simulink model "BPiKU_v3"  (R2018b)
settings: Solver=ode23t  StartTime=0.0  StopTime=6  RelTol=1e-6
undefined symbols (not defined in the file): Cdc, i_kt_int, i_kt_p, LdM, Lout, PointsVAH_I, PointsVAH_U, Rd, RdM, sigbuilder_block, u_k_int, u_k_p
libraries: powerlib x45, simulink x7, powerlib_meascontrol x3
settings Model: SimulationMode=accelerator  Creator=K2  LastModifiedBy=K2

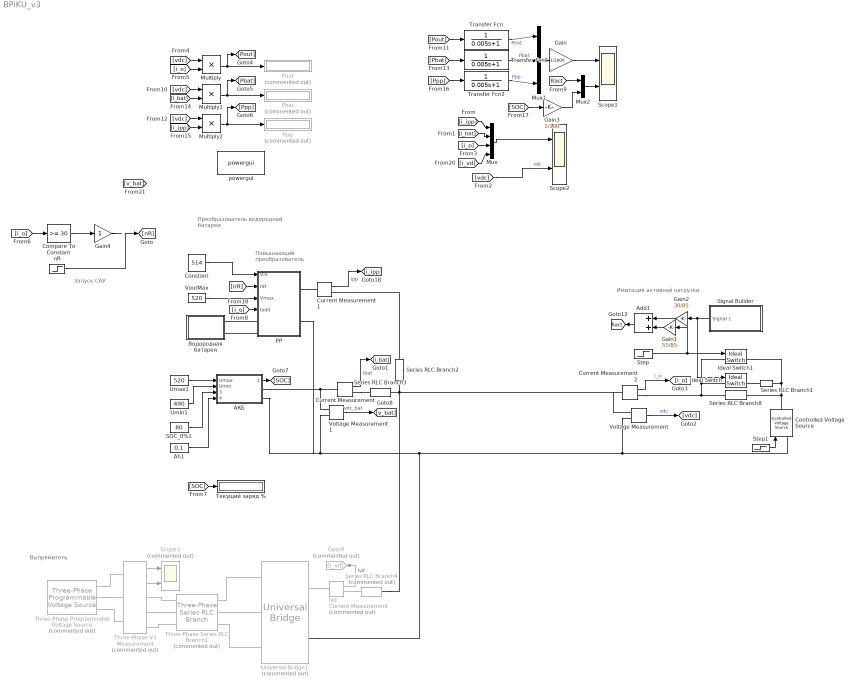
== system BPiKU_v3 ==
  note: Повышающий
      | преобразователь
  note: Имитация активной нагрузки
  note: Преобразователь водородной батареи
  note: Запуск САУ
  note: Выпрямитель
  Add1 : Sum
  Ah1 : Constant  Value=0.1
  Compare To Constant : simulink/Logic and Bit Operations/Compare To Constant  relop=>=  const=30  OutDataTypeStr=boolean
  Constant : Constant  Value=514
  Controlled Voltage Source : powerlib/Electrical Sources/Controlled Voltage Source  Initialize=on  Source_Type=AC  Amplitude=0  Phase=0  Frequency=0  Measurements=None
  Current Measurement : powerlib/Measurements/Current Measurement  PhasorSimulation=off  OutputType=Complex  PSBequivalent=0
  Current Measurement1 : powerlib/Measurements/Current Measurement  PhasorSimulation=off  OutputType=Complex  PSBequivalent=0
  Current Measurement2 : powerlib/Measurements/Current Measurement  PhasorSimulation=off  OutputType=Complex  PSBequivalent=0
  Gain : Gain  Gain=1/1000
  Gain1 : Gain  Gain=55/85
  Gain2 : Gain  Gain=30/85
  Gain3 : Gain  Gain=1/100
  Gain4 : Gain  OutDataTypeStr=double
  Goto9 : Goto  Commented=on  GotoTag=i_vd
  Ideal Switch : powerlib/Power Electronics/Ideal Switch  Ron=510*510/30000  Lon=0  IC=0  Rs=1e5  Cs=inf  Measurements=on
  Ideal Switch1 : powerlib/Power Electronics/Ideal Switch  Ron=550*550/45000  Lon=0  IC=0  Rs=1e5  Cs=inf  Measurements=on
  Multiply : Product
  Multiply1 : Product
  Multiply2 : Product
  Mux : Mux
  Mux1 : Mux  Inputs=3
  Mux2 : Mux  Inputs=2
  PP : Subsystem
  Pbat : Display  Commented=on
      settings: Format=bank
  Pout : Display  Commented=on
      settings: Format=bank
  Ppp : Display  Commented=on
      settings: Format=bank
  SOC_0%1 : Constant  Value=80
  Scope1 : Scope  NumInputPorts=2
  Scope2 : Scope  NumInputPorts=2
  Scope3 : Scope  Commented=on  NumInputPorts=2
  Series RLC Branch1 : powerlib/Elements/Series RLC Branch  LConnTagsString=__new0  RConnTagsString=__new0  BranchType=L  Resistance=550/130  Inductance=10e-3  SetiL0=off  InitialCurrent=0  Capacitance=1000e-6  Setx0=off  InitialVoltage=0  Measurements=None
  Series RLC Branch2 : powerlib/Elements/Series RLC Branch  LConnTagsString=__new0  RConnTagsString=__new0  BranchType=R  Resistance=0.01  Inductance=10e-6  SetiL0=off  InitialCurrent=0  Capacitance=1000e-6  Setx0=off  InitialVoltage=0  Measurements=None
  Series RLC Branch3 : powerlib/Elements/Series RLC Branch  LConnTagsString=__new0  RConnTagsString=__new0  BranchType=R  Resistance=0.01  Inductance=10e-6  SetiL0=off  InitialCurrent=0  Capacitance=1000e-6  Setx0=off  InitialVoltage=0  Measurements=None
  Series RLC Branch4 : powerlib/Elements/Series RLC Branch  Commented=on  LConnTagsString=__new0  RConnTagsString=__new0  BranchType=R  Resistance=0.01  Inductance=10e-6  SetiL0=off  InitialCurrent=0  Capacitance=1000e-6  Setx0=off  InitialVoltage=0  Measurements=None
  Series RLC Branch8 : powerlib/Elements/Series RLC Branch  LConnTagsString=__new0  RConnTagsString=__new0  BranchType=Open circuit  Resistance=550/130  Inductance=10e-6  SetiL0=off  InitialCurrent=0  Capacitance=1000e-6  Setx0=off  InitialVoltage=0  Measurements=None
  Signal Builder : Subsystem  Tag=STV Subsys  LoadFcn=sigbuilder_block('load');  StartFcn=sigbuilder_block('start');  StopFcn=sigbuilder_block('stop');  ClipboardFcn=sigbuilder_block('clipboard');  mask(Sigbuilder block){tuvar=[0:10]}
      mask help: Simulink:masks:SigbuilderBlock_MD
      mask init:
      | if ~strcmp(get_param(bdroot(gcbh),'SimulationStatus'),'stopped') tuvar = sigbuilder_block('maskInit'); end
      settings: CopyFcn=sigbuilder_block('copy');  DeleteFcn=sigbuilder_block('delete');  ModelCloseFcn=sigbuilder_block('modelClose');  PreSaveFcn=sigbuilder_block('preSave');  PauseFcn=sigbuilder_block('pause');  ContinueFcn=sigbuilder_block('continue');  NameChangeFcn=sigbuilder_block('namechange');  OpenFcn=sigbuilder_block('open',[193.5 84.75 550.5 399.75 ]);  CloseFcn=sigbuilder_block('close');
      mask Display: plot(0, 0, 100, 100,[2, 2, 32, 32, 2], [68, 8, 8, 68, 68],[32, 2], [38, 38], [32, 19, 2],[53, 60, 44], [32, 17, 17, 2],[16, 16, 31, 31]);txt = getActiveGroup(gcbh);text(2, 100, txt,'verticalAlignment', 'top');
  Step : Step  Time=4  SampleTime=0
  Step1 : Step  Time=3.5  After=800*0  SampleTime=0
  Three-Phase Programmable Voltage Source : powerlib/Electrical Sources/Three-Phase Programmable Voltage Source  Commented=on  PositiveSequence="[400  0 50]"  VariationEntity=None  VariationType=Table of time-amplitude pairs  VariationTypeAlt=Step  VariationStep=0.5  VariationRate=10  VariationMagnitude=0.3  VariationFrequency=2  VariationTiming=[1 2]  VariationPhaseA=off  Amplitudes=[1 0.8 1.2 1.0]  TimeValues=[0 0.1 0.15 0.2]  HarmonicGeneration=off  HarmonicA=[3 0.2 -25 0]  HarmonicB=[2 0.15 35 2]  Timing="[0.05  3]"  BusType=swing  Pref=0  Qref=0  Qmin=-inf  Qmax=inf
  Three-Phase Series RLC Branch1 : powerlib/Elements/Three-Phase Series RLC Branch  Commented=on  LConnTagsString=A|B|C  RConnTagsString=A|B|C  BranchType=RL  Resistance=0.001  Inductance=250e-6  Capacitance=105e-6  Measurements=None
  Three-Phase V-I Measurement : powerlib/Measurements/Three-Phase V-I Measurement  Commented=on  VoltageMeasurement=phase-to-phase  SetLabelV=off  LabelV=Vabc  Vpu=off  VpuLL=off  CurrentMeasurement=yes  SetLabelI=off  LabelI=Iabc  Ipu=off  Pbase=100e6  Vbase=500e3  OutputType=Complex  PhasorSimulation=off  PSBequivalent=0
  Transfer Fcn : TransferFcn  Denominator=[0.005 1]
  Transfer Fcn1 : TransferFcn  Denominator=[0.005 1]
  Transfer Fcn2 : TransferFcn  Denominator=[0.005 1]
  Umax1 : Constant  Value=520
  Umin1 : Constant  Value=490
  Universal Bridge1 : powerlib/Power Electronics/Universal Bridge  Commented=on  Arms=3  SnubberResistance=1e5  SnubberCapacitance=inf  Device=Diodes  Ron=1e-3  Lon=0  ForwardVoltages="[  0  0  ]"  ForwardVoltage=0  GTOparameters=[ 10e-6 , 20e-6 ]  IGBTparameters=[ 1e-6 , 2e-6 ]  Measurements=None  Measurements_2=None  converterType=Rectifier
  Voltage Measurement : powerlib/Measurements/Voltage Measurement  PhasorSimulation=off  OutputType=Complex  PSBequivalent=0
  Voltage Measurement1 : powerlib/Measurements/Voltage Measurement  PhasorSimulation=off  OutputType=Complex  PSBequivalent=0
  VoutMax : Constant  Value=520  SampleTime=0
  ivd : powerlib/Measurements/Current Measurement  Commented=on  PhasorSimulation=off  OutputType=Complex  PSBequivalent=0
  nR : Step  Time=0  SampleTime=1.5/freq/2
  powergui : powerlib/powergui  Priority=1  SimulationMode=Discrete  SampleTime=1e-6  frequency=60  Iterations=50  frequencyindice=0  Pbase=100e6  ErrMax=1e-4  UnitsV=kV  UnitsW=MW  buscounter=0  FunctionMessages=off  echomessages=off  EnableUseOfTLC=off  CurrentSourceSwitches=off  DisableSnubberDevices=off  DisableRonSwitches=off  DisableVfSwitches=off  DisplayEquations=off  SolverType=Tustin  Interpol=off  ExternalGateDelay=off  methode=off  Ts=100  x0status=blocks  SPID=off  SwTol=0  HookPort=off  RestoreLinks=warning  ResistiveCurrentMeasurement=off  Frange=[0:2:500]  Ylog=off  Xlog=on  ShowGrid=off  save=off  variable=ZData  structure=0  ZoomFFT=off  StartTime=0.0  cycles=1  DisplayStyle=1  fundamental=60  FreqAxis=off  MaxFrequency=1000  frequencyindicesteady=1  RmsSteady=1  display=off
  АКБ : Subsystem
  Водородная батарея : Subsystem
  Текущий заряд % : Display
      settings: Format=bank
  tag scope: Ract=global
  wires:
  Signal Builder/1(Signal 1) -> Gain2/1, Ideal Switch/1
  VoutMax/1 -> PP/3(Vmax)
  [nR] -> PP/2(nR)
  Current Measurement1/1 -> [i_ipp]  "ipp"
  [vdc] -> Scope2/2  "vdc"
  Mux/1 -> Scope2/1
  [i_ipp] -> Mux/1
  Current Measurement/1 -> [i_bat]  "ibat"
  [i_bat] -> Mux/2
  Voltage Measurement/1 -> [vdc]  "vdc"
  Current Measurement2/1 -> [i_o]  "i_o"
  [i_o] -> Mux/3
  [vdc] -> Multiply/1
  [i_o] -> Multiply/2
  Multiply/1 -> [Pout], Pout/1
  Step/1 -> Ideal Switch1/1, Gain1/1
  [Ppp] -> Transfer Fcn2/1
  [Pbat] -> Transfer Fcn1/1
  [Pout] -> Transfer Fcn/1
  [vdc] -> Multiply1/1
  [i_bat] -> Multiply1/2
  [i_ipp] -> Multiply2/2
  [vdc] -> Multiply2/1
  Multiply1/1 -> [Pbat], Pbat/1
  Multiply2/1 -> [Ppp], Ppp/1
  Transfer Fcn/1 -> Mux1/1  "Pout"
  Transfer Fcn1/1 -> Mux1/2  "Pbat"
  Transfer Fcn2/1 -> Mux1/3  "Ppp"
  АКБ/1(CurSOC%) -> [SOC]
  [SOC] -> Текущий заряд %/1
  Constant/1 -> PP/1(Vin)
  Mux1/1 -> Gain/1
  [Ract] -> Mux2/1
  Gain/1 -> Scope1/1
  Add1/1 -> [Ract]
  Gain1/1 -> Add1/2
  Gain2/1 -> Add1/1
  Mux2/1 -> Scope1/2
  [SOC] -> Gain3/1
  Gain3/1 -> Mux2/2
  Compare To Constant/1 -> Gain4/1
  Three-Phase V-I Measurement/2 -> Scope3/2
  Three-Phase V-I Measurement/1 -> Scope3/1
  ivd/1 -> Goto9/1  "ivd"
  [i_vd] -> Mux/4
  Step1/1 -> Controlled Voltage Source/1
  SOC_0%1/1 -> АКБ/3(InitSOC%)
  Umax1/1 -> АКБ/1(Umax)
  Ah1/1 -> АКБ/4(CapMaxAh)
  Umin1/1 -> АКБ/2(Umin)
  [i_o] -> Compare To Constant/1
  nR/1 -> [nR]
  Gain4/1 -> ?
  [i_o] -> PP/4(Iadd)
  Voltage Measurement1/1 -> [v_bat]  "vdc_bat"
  connections:
  Ideal Switch/RConn1 -- Series RLC Branch1/LConn1
  PP/LConn2 -- Водородная батарея/RConn2
  PP/LConn1 -- Водородная батарея/RConn1
  PP/RConn1 -- Current Measurement1/LConn1
  Series RLC Branch8/LConn1 -- Current Measurement2/RConn1 -- Ideal Switch/LConn1 -- Ideal Switch1/LConn1
  Series RLC Branch2/LConn1 -- Current Measurement1/RConn1
  Current Measurement/RConn1 -- Series RLC Branch3/RConn1
  Voltage Measurement/LConn2 -- Voltage Measurement1/LConn2 -- PP/RConn2 -- АКБ/RConn2 -- Universal Bridge1/RConn2 -- Controlled Voltage Source/LConn1
  Universal Bridge1/LConn3 -- Three-Phase Series RLC Branch1/RConn3
  Three-Phase Series RLC Branch1/RConn2 -- Universal Bridge1/LConn2
  Three-Phase Programmable Voltage Source/RConn2 -- Three-Phase V-I Measurement/LConn2
  Three-Phase Programmable Voltage Source/RConn3 -- Three-Phase V-I Measurement/LConn3
  Universal Bridge1/LConn1 -- Three-Phase Series RLC Branch1/RConn1
  Three-Phase Programmable Voltage Source/RConn1 -- Three-Phase V-I Measurement/LConn1
  ivd/LConn1 -- Universal Bridge1/RConn1
  Series RLC Branch4/RConn1 -- ivd/RConn1
  Series RLC Branch3/LConn1 -- Current Measurement2/LConn1 -- Voltage Measurement/LConn1 -- Series RLC Branch4/LConn1 -- Series RLC Branch2/RConn1
  Three-Phase Series RLC Branch1/LConn3 -- Three-Phase V-I Measurement/RConn3
  Three-Phase Series RLC Branch1/LConn2 -- Three-Phase V-I Measurement/RConn2
  Three-Phase Series RLC Branch1/LConn1 -- Three-Phase V-I Measurement/RConn1
  Ideal Switch1/RConn1 -- Series RLC Branch1/RConn1 -- Series RLC Branch8/RConn1 -- Controlled Voltage Source/RConn1
  АКБ/RConn1 -- Voltage Measurement1/LConn1 -- Current Measurement/LConn1

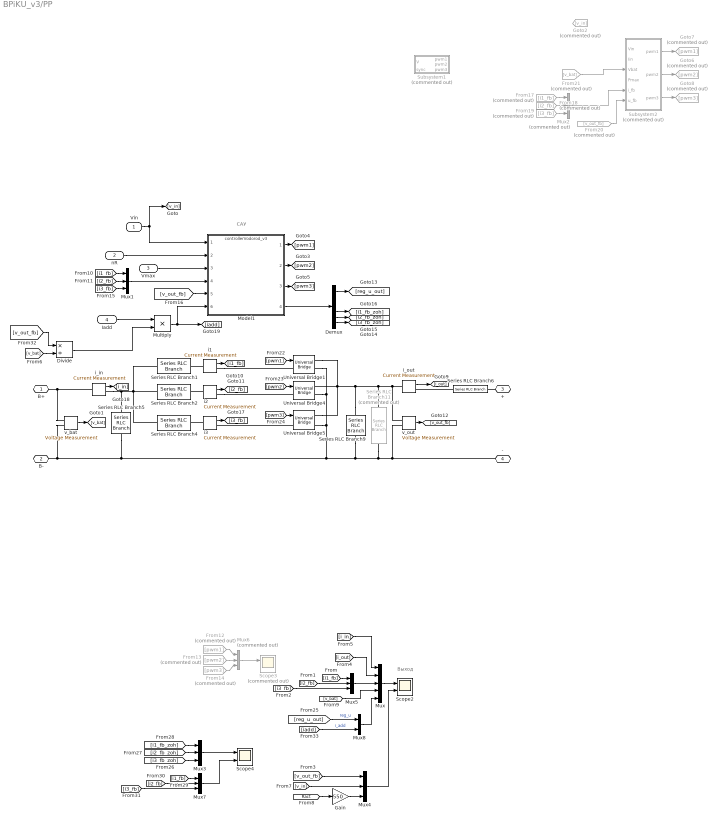
== system BPiKU_v3/PP ==
  note: САУ
  note: Выход
  Vin : Inport
  nR : Inport  Port=2
  Vmax : Inport  Port=3
  Iadd : Inport  Port=4
  Demux : Demux  Outputs=7
  Divide : Product  Inputs=*/
  From12 : From  Commented=on  GotoTag=pwm1
  From13 : From  Commented=on  GotoTag=pwm2
  From14 : From  Commented=on  GotoTag=pwm3
  From17 : From  Commented=on  GotoTag=i1_fb
  From18 : From  Commented=on  GotoTag=i2_fb
  From19 : From  Commented=on  GotoTag=i3_fb
  From20 : From  Commented=on  GotoTag=v_out_fb
  From21 : From  Commented=on  GotoTag=v_bat
  Gain : Gain  Gain=550
  Goto2 : Goto  Commented=on  GotoTag=v_in
  Goto6 : Goto  Commented=on  GotoTag=pwm2
  Goto7 : Goto  Commented=on  GotoTag=pwm1
  Goto8 : Goto  Commented=on  GotoTag=pwm3
  Model1 : ModelReference  ModelNameDialog=controllerVodorod_v3.slx  SimulationMode=Normal  ModelReferenceVersion=1.32
  Multiply : Product
  Mux : Mux  Inputs=5
  Mux{1,3..5,7} (5 alike) : Mux  Inputs=3
  Mux2 : Mux  Commented=on  Inputs=3
  Mux6 : Mux  Commented=on  Inputs=3
  Mux8 : Mux  Inputs=2
  Scope2 : Scope  NumInputPorts=2
  Scope3 : Scope  Commented=on  NumInputPorts=2
  Scope4 : Scope  NumInputPorts=2
  Series RLC Branch1 : powerlib/Elements/Series RLC Branch  LConnTagsString=__new0  RConnTagsString=__new0  BranchType=RL  Resistance=RdM(1)  Inductance=LdM(1)  SetiL0=off  InitialCurrent=0  Capacitance=100e-6  Setx0=off  InitialVoltage=0  Measurements=None
  Series RLC Branch11 : powerlib/Elements/Series RLC Branch  Commented=on  LConnTagsString=__new0  RConnTagsString=__new0  BranchType=Open circuit  Resistance=2000  Inductance=50e-6  SetiL0=off  InitialCurrent=0  Capacitance=100e-6  Setx0=off  InitialVoltage=0  Measurements=None
  Series RLC Branch2 : powerlib/Elements/Series RLC Branch  LConnTagsString=__new0  RConnTagsString=__new0  BranchType=RL  Resistance=RdM(2)  Inductance=LdM(2)  SetiL0=off  InitialCurrent=0  Capacitance=100e-6  Setx0=off  InitialVoltage=0  Measurements=None
  Series RLC Branch4 : powerlib/Elements/Series RLC Branch  LConnTagsString=__new0  RConnTagsString=__new0  BranchType=RL  Resistance=RdM(3)  Inductance=LdM(3)  SetiL0=off  InitialCurrent=0  Capacitance=100e-6  Setx0=off  InitialVoltage=0  Measurements=None
  Series RLC Branch5 : powerlib/Elements/Series RLC Branch  LConnTagsString=__new0  RConnTagsString=__new0  BranchType=RC  Resistance=0.001  Inductance=50e-6  SetiL0=off  InitialCurrent=0  Capacitance=8000e-6  Setx0=on  InitialVoltage=340  Measurements=None
  Series RLC Branch6 : powerlib/Elements/Series RLC Branch  LConnTagsString=__new0  RConnTagsString=__new0  BranchType=RL  Resistance=Rd  Inductance=Lout  SetiL0=off  InitialCurrent=0  Capacitance=1e-6  Setx0=off  InitialVoltage=0  Measurements=None
  Series RLC Branch9 : powerlib/Elements/Series RLC Branch  LConnTagsString=__new0  RConnTagsString=__new0  BranchType=C  Resistance=0.0001  Inductance=50e-6  SetiL0=off  InitialCurrent=0  Capacitance=Cdc  Setx0=on  InitialVoltage=510  Measurements=None
  Subsystem1 : Subsystem  Commented=on
  Subsystem2 : Subsystem  Commented=on
  Universal Bridge1 : powerlib/Power Electronics/Universal Bridge  Arms=1  SnubberResistance=1e5  SnubberCapacitance=inf  Device=MOSFET / Diodes  Ron=1e-3  Lon=0  ForwardVoltages="[  2  2  ]"  ForwardVoltage=0  GTOparameters=[ 10e-6 , 20e-6 ]  IGBTparameters=[ 1e-6 , 2e-6 ]  Measurements=None  Measurements_2=None  converterType=Rectifier
  Universal Bridge4 : powerlib/Power Electronics/Universal Bridge  Arms=1  SnubberResistance=1e5  SnubberCapacitance=inf  Device=MOSFET / Diodes  Ron=1e-3  Lon=0  ForwardVoltages="[  2  2  ]"  ForwardVoltage=0  GTOparameters=[ 10e-6 , 20e-6 ]  IGBTparameters=[ 1e-6 , 2e-6 ]  Measurements=None  Measurements_2=None  converterType=Rectifier
  Universal Bridge5 : powerlib/Power Electronics/Universal Bridge  Arms=1  SnubberResistance=1e5  SnubberCapacitance=inf  Device=MOSFET / Diodes  Ron=1e-3  Lon=0  ForwardVoltages="[  2  2  ]"  ForwardVoltage=0  GTOparameters=[ 10e-6 , 20e-6 ]  IGBTparameters=[ 1e-6 , 2e-6 ]  Measurements=None  Measurements_2=None  converterType=Rectifier
  i1 : powerlib/Measurements/Current Measurement  PhasorSimulation=off  OutputType=Complex  PSBequivalent=0
  i2 : powerlib/Measurements/Current Measurement  PhasorSimulation=off  OutputType=Complex  PSBequivalent=0
  i3 : powerlib/Measurements/Current Measurement  PhasorSimulation=off  OutputType=Complex  PSBequivalent=0
  i_in : powerlib/Measurements/Current Measurement  PhasorSimulation=off  OutputType=Complex  PSBequivalent=0
  i_out : powerlib/Measurements/Current Measurement  PhasorSimulation=off  OutputType=Complex  PSBequivalent=0
  v_bat : powerlib/Measurements/Voltage Measurement  PhasorSimulation=off  OutputType=Complex  PSBequivalent=0
  v_out : powerlib/Measurements/Voltage Measurement  PhasorSimulation=off  OutputType=Complex  PSBequivalent=0
  B+ : PMIOPort  Side=Left
  B- : PMIOPort  Port=2  Side=Left
  + : PMIOPort  Port=3  Side=Right
  - : PMIOPort  Port=4  Side=Right
  wires:
  From14/1 -> Mux6/3
  From12/1 -> Mux6/1
  [v_in] -> Mux4/2
  Mux5/1 -> Mux/3
  [v_out_fb] -> Mux4/1
  Mux/1 -> Scope2/1
  [i_in] -> Mux/1
  [i_out] -> Mux/2
  [i1_fb] -> Mux5/1
  From13/1 -> Mux6/2
  Mux6/1 -> Scope3/1
  [i2_fb] -> Mux5/2
  Mux4/1 -> Scope2/2
  [i3_fb] -> Mux5/3
  Model1/2 -> [pwm2]
  Model1/1 -> [pwm1]
  Vin/1 -> Model1/1, [v_in]
  Model1/3 -> [pwm3]
  nR/1 -> Model1/2
  Vmax/1 -> Model1/3
  [Ract] -> Gain/1
  Gain/1 -> Mux4/3
  [v_out_fb] -> Model1/5
  [v_bat] -> Mux/4
  [i2_fb] -> Mux1/2
  [i3_fb] -> Mux1/3
  [i1_fb] -> Mux1/1
  Mux1/1 -> Model1/4
  i1/1 -> [i1_fb]
  i_in/1 -> [i_in]
  i_out/1 -> [i_out]
  i2/1 -> [i2_fb]
  v_bat/1 -> [v_bat]
  [pwm1] -> Universal Bridge1/1
  [pwm2] -> Universal Bridge4/1
  v_out/1 -> [v_out_fb]
  [pwm3] -> Universal Bridge5/1
  i3/1 -> [i3_fb]
  From20/1 -> Subsystem2/6(u_fb)
  From21/1 -> Subsystem2/3(Vbat)
  From18/1 -> Mux2/2
  Mux2/1 -> Subsystem2/5(i_fb)
  From17/1 -> Mux2/1
  ? -> Subsystem2/4(Pmax)
  From19/1 -> Mux2/3
  Subsystem2/2(pwm2) -> Goto6/1
  Subsystem2/1(pwm1) -> Goto7/1
  Subsystem2/3(pwm3) -> Goto8/1
  ? -> Subsystem2/2(Iin)
  ? -> Goto2/1, Subsystem2/1(Vin)
  Model1/4 -> Demux/1
  Demux/1 -> [reg_u_out]
  Mux8/1 -> Mux/5
  Demux/7 -> [i3_fb_zoh]
  Demux/6 -> [i2_fb_zoh]
  Demux/5 -> [i1_fb_zoh]
  [i2_fb_zoh] -> Mux3/2
  [i1_fb_zoh] -> Mux3/1
  [i3_fb_zoh] -> Mux3/3
  Mux3/1 -> Scope4/1
  [i2_fb] -> Mux7/2
  [i3_fb] -> Mux7/3
  Mux7/1 -> Scope4/2
  [i1_fb] -> Mux7/1
  Multiply/1 -> [iadd], Model1/6
  Iadd/1 -> Multiply/1
  [v_bat] -> Divide/2
  [v_out_fb] -> Divide/1
  Divide/1 -> Multiply/2
  [reg_u_out] -> Mux8/1  "reg_u"
  [iadd] -> Mux8/2  "i_add"
  connections:
  Series RLC Branch9/LConn1 -- Series RLC Branch11/LConn1 -- v_out/LConn1 -- i_out/LConn1 -- Universal Bridge5/RConn1 -- Universal Bridge1/RConn1 -- Universal Bridge4/RConn1
  v_bat/LConn2 -- B-/RConn1 -- Series RLC Branch5/RConn1 -- Universal Bridge5/RConn2 -- Universal Bridge1/RConn2 -- Universal Bridge4/RConn2 -- Series RLC Branch9/RConn1 -- Series RLC Branch11/RConn1 -- v_out/LConn2 -- -/RConn1
  Series RLC Branch1/LConn1 -- i_in/RConn1 -- Series RLC Branch5/LConn1 -- Series RLC Branch4/LConn1 -- Series RLC Branch2/LConn1
  v_bat/LConn1 -- B+/RConn1 -- i_in/LConn1
  i2/LConn1 -- Series RLC Branch2/RConn1
  +/RConn1 -- Series RLC Branch6/LConn1
  i1/RConn1 -- Universal Bridge1/LConn1
  Series RLC Branch6/RConn1 -- i_out/RConn1
  i2/RConn1 -- Universal Bridge4/LConn1
  Universal Bridge5/LConn1 -- i3/RConn1
  i1/LConn1 -- Series RLC Branch1/RConn1
  i3/LConn1 -- Series RLC Branch4/RConn1

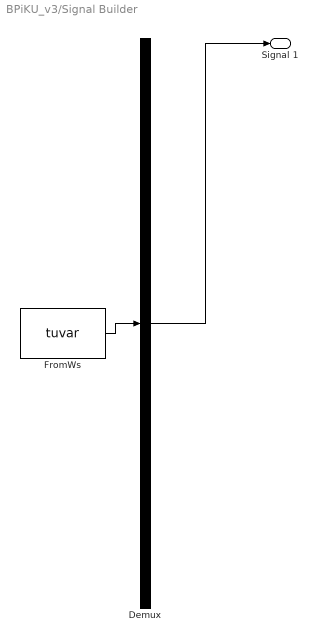
== system BPiKU_v3/Signal Builder ==
  Demux : Demux  Tag=STV Demux  Outputs=1
  FromWs : FromWorkspace  Tag=STV FromWs  VariableName=tuvar  SampleTime=0
      SigBuilderData=|
      | common.afterFinalStr = 'Extrapolate'
      | common.sampleTime = 0
      | dataSet.timeRange = [0 10]
      | dataSet.name = 'Group 1'
      | sbobj.Groups.Name = 'Group 1'
      | sbobj.Groups.Signals.Name = 'Signal 1'
      | sbobj.Groups.Signals.XData = [0 0.02 0.1 0.1 0.17 0.17 0.55 0.55 2.02 2.02 2.07 2.07 2.49 2.49 2.62 2.62 2.87 2.87 3.8 3.8 4.06 4.06 6 10]
      | sbobj.Groups.Signals.YData = [0 0 0 1 1 0 0 1 1 0 0 1 1 0 0 1 1 0 0 1 1 0 0 0]
  Signal 1 : Outport  Tag=STV Outport
  wires:
  Demux/1 -> Signal 1/1
  FromWs/1 -> Demux/1

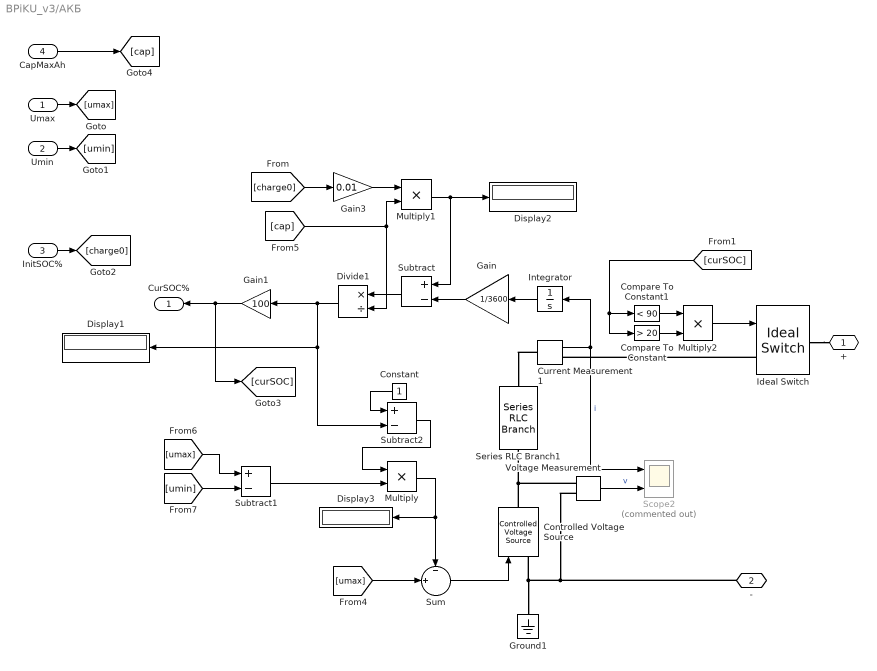
== system BPiKU_v3/АКБ ==
  Umax : Inport
  Umin : Inport  Port=2
  InitSOC% : Inport  Port=3
  CapMaxAh : Inport  Port=4
  Compare To Constant : simulink/Logic and Bit Operations/Compare To Constant  relop=>  const=20  OutDataTypeStr=boolean
  Compare To Constant1 : simulink/Logic and Bit Operations/Compare To Constant  relop=<  const=90  OutDataTypeStr=boolean
  Constant : Constant
  Controlled Voltage Source : powerlib/Electrical Sources/Controlled Voltage Source  Initialize=on  Source_Type=AC  Amplitude=0  Phase=0  Frequency=0  Measurements=None
  Current Measurement1 : powerlib/Measurements/Current Measurement  PhasorSimulation=off  OutputType=Complex  PSBequivalent=0
  Display1 : Display
  Display2 : Display
  Display3 : Display
  Divide1 : Product  Inputs=*/
  Gain : Gain  Gain=1/3600
  Gain1 : Gain  Gain=100
  Gain3 : Gain  Gain=0.01
  Ground1 : powerlib/Elements/Ground  LConnTagsString=a
  Ideal Switch : powerlib/Power Electronics/Ideal Switch  Ron=0.001  Lon=0  IC=0  Rs=1e5  Cs=inf  Measurements=off
  Integrator : Integrator
  Multiply : Product
  Multiply1 : Product
  Multiply2 : Product
  Scope2 : Scope  Commented=on  NumInputPorts=2
  Series RLC Branch1 : powerlib/Elements/Series RLC Branch  LConnTagsString=__new0  RConnTagsString=__new0  BranchType=R  Resistance=0.01  Inductance=10e-6  SetiL0=off  InitialCurrent=0  Capacitance=1000e-6  Setx0=off  InitialVoltage=0  Measurements=None
  Subtract : Sum  Inputs=+-
  Subtract1 : Sum  Inputs=+-
  Subtract2 : Sum  Inputs=+-
  Sum : Sum  Inputs=-|+||
  Voltage Measurement : powerlib/Measurements/Voltage Measurement  PhasorSimulation=off  OutputType=Complex  PSBequivalent=0
  + : PMIOPort  Side=Right
  - : PMIOPort  Port=2  Side=Right
  CurSOC% : Outport
  wires:
  [umax] -> Sum/2
  Sum/1 -> Controlled Voltage Source/1
  Integrator/1 -> Gain/1
  Voltage Measurement/1 -> Scope2/2  "v"
  Current Measurement1/1 -> Integrator/1, Scope2/1  "i"
  Divide1/1 -> Subtract2/2, Display1/1, Gain1/1
  Umax/1 -> [umax]
  Umin/1 -> [umin]
  InitSOC%/1 -> [charge0]
  CapMaxAh/1 -> [cap]
  [charge0] -> Gain3/1
  Gain3/1 -> Multiply1/1
  [cap] -> Divide1/2, Multiply1/2
  Multiply1/1 -> Subtract/1, Display2/1
  Gain/1 -> Subtract/2
  Subtract/1 -> Divide1/1
  [umax] -> Subtract1/1
  [umin] -> Subtract1/2
  Subtract1/1 -> Multiply/2
  Multiply/1 -> Display3/1, Sum/1
  Constant/1 -> Subtract2/1
  Subtract2/1 -> Multiply/1
  [curSOC] -> Compare To Constant1/1, Compare To Constant/1
  Compare To Constant/1 -> Multiply2/2
  Gain1/1 -> [curSOC], CurSOC%/1
  Compare To Constant1/1 -> Multiply2/1
  Multiply2/1 -> Ideal Switch/1
  connections:
  -/RConn1 -- Ground1/LConn1 -- Controlled Voltage Source/LConn1 -- Voltage Measurement/LConn2
  Current Measurement1/LConn1 -- Series RLC Branch1/LConn1
  Controlled Voltage Source/RConn1 -- Series RLC Branch1/RConn1 -- Voltage Measurement/LConn1
  Ideal Switch/LConn1 -- Current Measurement1/RConn1
  Ideal Switch/RConn1 -- +/RConn1

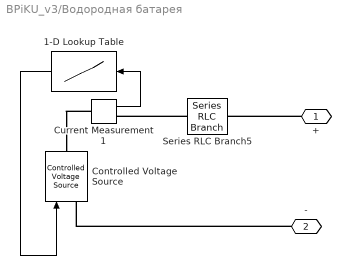
== system BPiKU_v3/Водородная батарея ==
  1-D Lookup Table : Lookup_n-D  NumberOfTableDimensions=1  BreakpointsForDimension1=PointsVAH_I  Table=PointsVAH_U  InternalRulePriority=Speed  RndMeth=Simplest  InputSameDT=on
  Controlled Voltage Source : powerlib/Electrical Sources/Controlled Voltage Source  Initialize=on  Source_Type=AC  Amplitude=0  Phase=0  Frequency=0  Measurements=None
  Current Measurement1 : powerlib/Measurements/Current Measurement  PhasorSimulation=off  OutputType=Complex  PSBequivalent=0
  Series RLC Branch5 : powerlib/Elements/Series RLC Branch  LConnTagsString=__new0  RConnTagsString=__new0  BranchType=R  Resistance=0.1  Inductance=50e-6  SetiL0=off  InitialCurrent=0  Capacitance=8000e-6  Setx0=on  InitialVoltage=340  Measurements=None
  + : PMIOPort  Side=Right
  - : PMIOPort  Port=2  Side=Right
  wires:
  1-D Lookup Table/1 -> Controlled Voltage Source/1
  Current Measurement1/1 -> 1-D Lookup Table/1
  connections:
  -/RConn1 -- Controlled Voltage Source/LConn1
  Current Measurement1/LConn1 -- Controlled Voltage Source/RConn1
  Series RLC Branch5/LConn1 -- Current Measurement1/RConn1
  +/RConn1 -- Series RLC Branch5/RConn1

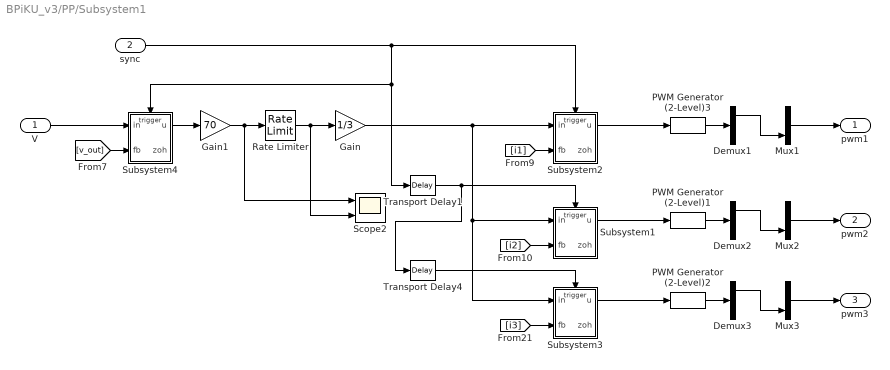
== system BPiKU_v3/PP/Subsystem1 ==
  V : Inport
  sync : Inport  Port=2
  Demux1 : Demux  Outputs=2
  Demux2 : Demux  Outputs=2
  Demux3 : Demux  Outputs=2
  Gain : Gain  Gain=1/3
  Gain1 : Gain  Gain=70
  Mux1 : Mux  Inputs=2
  Mux2 : Mux  Inputs=2
  Mux3 : Mux  Inputs=2
  PWM Generator (2-Level)1 : powerlib_meascontrol/Pulse & Signal Generators/PWM Generator (2-Level)  ModulatorType=Single-phase half-bridge (2 pulses)  ModulatorMode=Unsynchronized  Fc=freq  Pc=120  nF=1  MinMax="[0.001  1 ]"  SamplingTechnique=Natural  ModulatingSignals=off  m=0.8  Freq=60  Phase=0  Ts=0  ShowCarrierOutport=off
      settings: SourceProductName=Simscape Power Systems
  PWM Generator (2-Level)2 : powerlib_meascontrol/Pulse & Signal Generators/PWM Generator (2-Level)  ModulatorType=Single-phase half-bridge (2 pulses)  ModulatorMode=Unsynchronized  Fc=freq  Pc=-120  nF=1  MinMax="[0.001  1 ]"  SamplingTechnique=Natural  ModulatingSignals=off  m=0.8  Freq=60  Phase=0  Ts=0  ShowCarrierOutport=off
      settings: SourceProductName=Simscape Power Systems
  PWM Generator (2-Level)3 : powerlib_meascontrol/Pulse & Signal Generators/PWM Generator (2-Level)  ModulatorType=Single-phase half-bridge (2 pulses)  ModulatorMode=Unsynchronized  Fc=freq  Pc=0  nF=1  MinMax="[0.001  1 ]"  SamplingTechnique=Natural  ModulatingSignals=off  m=0.8  Freq=60  Phase=0  Ts=0  ShowCarrierOutport=off
      settings: SourceProductName=Simscape Power Systems
  Rate Limiter : RateLimiter  RisingSlewLimit=15  FallingSlewLimit=-15  SampleTimeMode=inherited
  Scope2 : Scope  NumInputPorts=2
  Subsystem1 : Subsystem
  Subsystem2 : Subsystem
  Subsystem3 : Subsystem
  Subsystem4 : Subsystem
  Transport Delay1 : TransportDelay  DelayTime=1/freq/2/3
  Transport Delay4 : TransportDelay  DelayTime=1/freq/2/3
  pwm1 : Outport
  pwm2 : Outport  Port=2
  pwm3 : Outport  Port=3
  wires:
  [i2] -> Subsystem1/2(fb)
  [i3] -> Subsystem3/2(fb)
  sync/1 -> Subsystem4/Trigger, Transport Delay1/1, Subsystem2/Trigger
  Transport Delay1/1 -> Subsystem1/Trigger, Transport Delay4/1
  Transport Delay4/1 -> Subsystem3/Trigger
  Mux1/1 -> pwm1/1
  Subsystem2/1(u) -> PWM Generator (2-Level)3/1
  PWM Generator (2-Level)3/1 -> Demux1/1
  Demux1/1 -> Mux1/2
  V/1 -> Subsystem4/1(in)
  [i1] -> Subsystem2/2(fb)
  Gain/1 -> Subsystem3/1(in), Subsystem1/1(in), Subsystem2/1(in)
  PWM Generator (2-Level)2/1 -> Demux3/1
  PWM Generator (2-Level)1/1 -> Demux2/1
  Mux2/1 -> pwm2/1
  [v_out] -> Subsystem4/2(fb)
  Subsystem3/1(u) -> PWM Generator (2-Level)2/1
  Demux2/1 -> Mux2/2
  Demux3/1 -> Mux3/2
  Subsystem1/1(u) -> PWM Generator (2-Level)1/1
  Subsystem4/1(u) -> Gain1/1
  Mux3/1 -> pwm3/1
  Rate Limiter/1 -> Scope2/2, Gain/1
  Gain1/1 -> Scope2/1, Rate Limiter/1

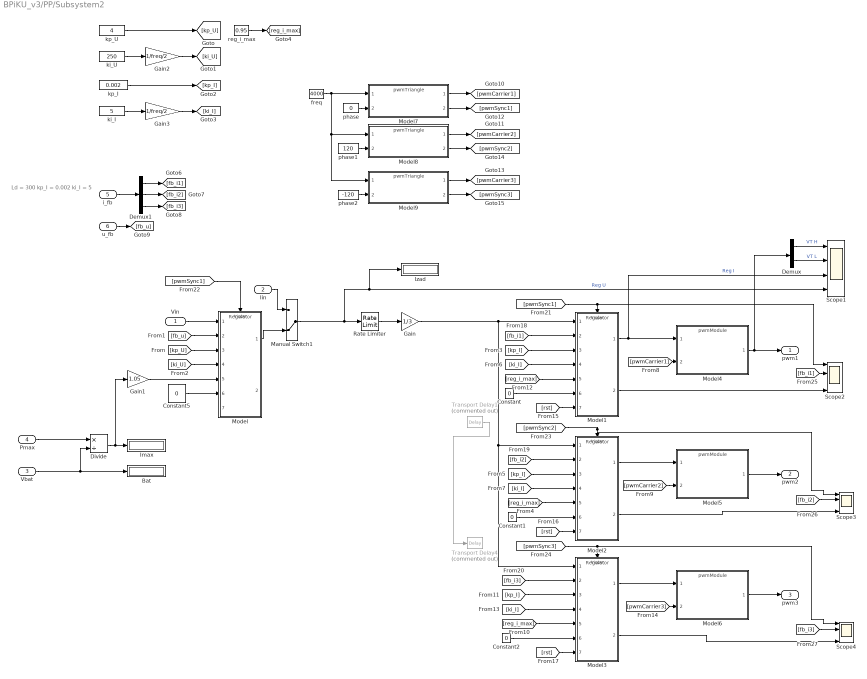
== system BPiKU_v3/PP/Subsystem2 ==
  note: Ld = 300
      | kp_I = 0.002
      | ki_I = 5
  Vin : Inport
  Iin : Inport  Port=2
  Vbat : Inport  Port=3
  Pmax : Inport  Port=4
  i_fb : Inport  Port=5
  u_fb : Inport  Port=6
  Bat : Display
      settings: Format=bank
  Constant{,1..2,5} (4 alike) : Constant  Value=0
  Demux : Demux  Outputs=2
  Demux1 : Demux  Outputs=3
  Divide : Product  Inputs=*/
  Gain : Gain  Gain=1/3
  Gain1 : Gain  Gain=1.05
  Gain2 : Gain  Gain=1/freq/2
  Gain3 : Gain  Gain=1/freq/2
  Imax : Display
      settings: Format=bank
  Izad : Display
      settings: Format=bank
  Manual Switch1 : ManualSwitch  CurrentSetting=0
  Model{,1..3} (4 alike) : ModelReference  ModelNameDialog=Regulator.slx  SimulationMode=Normal  ModelReferenceVersion=1.38  TriggerPortName=Trigger  TriggerPortTriggerType=either
  Model4 : ModelReference  ModelNameDialog=pwmModule.slx  SimulationMode=Normal  ModelReferenceVersion=1.2
  Model5 : ModelReference  ModelNameDialog=pwmModule.slx  SimulationMode=Normal  ModelReferenceVersion=1.2
  Model6 : ModelReference  ModelNameDialog=pwmModule.slx  SimulationMode=Normal  ModelReferenceVersion=1.2
  Model7 : ModelReference  ModelNameDialog=pwmTriangle.slx  SimulationMode=Normal  ModelReferenceVersion=1.5
  Model8 : ModelReference  ModelNameDialog=pwmTriangle.slx  SimulationMode=Normal  ModelReferenceVersion=1.5
  Model9 : ModelReference  ModelNameDialog=pwmTriangle.slx  SimulationMode=Normal  ModelReferenceVersion=1.5
  Rate Limiter : RateLimiter  RisingSlewLimit=1000  FallingSlewLimit=-100000  SampleTimeMode=inherited
  Scope{1..4} (4 alike) : Scope  NumInputPorts=4
  Transport Delay1 : TransportDelay  Commented=on  DelayTime=1/freq/2/3
  Transport Delay4 : TransportDelay  Commented=on  DelayTime=1/freq/2/3
  freq : Constant  Value=4000
  ki_I : Constant  Value=5
  ki_U : Constant  Value=250
  kp_I : Constant  Value=0.002
  kp_U : Constant  Value=4
  phase : Constant  Value=0
  phase1 : Constant  Value=120
  phase2 : Constant  Value=-120
  reg_i_max : Constant  Value=0.95
  pwm1 : Outport
  pwm2 : Outport  Port=2
  pwm3 : Outport  Port=3
  wires:
  Transport Delay1/1 -> Transport Delay4/1
  Rate Limiter/1 -> Gain/1
  [fb_u] -> Model/2
  Divide/1 -> Gain1/1, Imax/1
  Model/1 -> Manual Switch1/2
  Pmax/1 -> Divide/1
  Vbat/1 -> Bat/1, Divide/2
  Vin/1 -> Model/1
  [reg_i_max] -> Model1/5
  [fb_i1] -> Model1/2
  Model5/1 -> pwm2/1
  Model6/1 -> pwm3/1
  Gain/1 -> Model3/1, Model2/1, Model1/1
  Model4/1 -> Demux/1, pwm1/1
  Demux/1 -> Scope1/1  "VT H"
  Demux/2 -> Scope1/2  "VT L"
  Model1/1 -> Scope1/3, Model4/1  "Reg I"
  Manual Switch1/1 -> Rate Limiter/1, Izad/1, Scope1/4  "Reg U"
  Constant5/1 -> Model/6
  kp_U/1 -> [kp_U]
  ki_U/1 -> Gain2/1
  [kp_U] -> Model/3
  [ki_U] -> Model/4
  kp_I/1 -> [kp_I]
  ki_I/1 -> Gain3/1
  [kp_I] -> Model1/3
  [ki_I] -> Model1/4
  reg_i_max/1 -> [reg_i_max]
  [kp_I] -> Model3/3
  [fb_i3] -> Model3/2
  [ki_I] -> Model3/4
  [reg_i_max] -> Model3/5
  [reg_i_max] -> Model2/5
  [kp_I] -> Model2/3
  [ki_I] -> Model2/4
  [fb_i2] -> Model2/2
  Constant/1 -> Model1/6
  Constant1/1 -> Model2/6
  Constant2/1 -> Model3/6
  [rst] -> Model1/7
  [rst] -> Model2/7
  [rst] -> Model3/7
  Gain2/1 -> [ki_U]
  Gain3/1 -> [ki_I]
  i_fb/1 -> Demux1/1
  Demux1/1 -> [fb_i1]
  Demux1/2 -> [fb_i2]
  Demux1/3 -> [fb_i3]
  u_fb/1 -> [fb_u]
  phase/1 -> Model7/2
  freq/1 -> Model8/1, Model9/1, Model7/1
  Model7/1 -> [pwmCarrier1]
  Model8/2 -> [pwmSync2]
  Model9/2 -> [pwmSync3]
  Model8/1 -> [pwmCarrier2]
  Model9/1 -> [pwmCarrier3]
  phase1/1 -> Model8/2
  Model7/2 -> [pwmSync1]
  phase2/1 -> Model9/2
  [pwmSync1] -> Model1/Trigger, Scope2/1
  [pwmCarrier1] -> Model4/2
  [pwmCarrier2] -> Model5/2
  Model2/1 -> Model5/1
  Model3/1 -> Model6/1
  [pwmCarrier3] -> Model6/2
  Gain1/1 -> Model/5
  Iin/1 -> Manual Switch1/1
  [pwmSync1] -> Model/Trigger
  Model1/2 -> Scope2/4
  [fb_i1] -> Scope2/2
  [fb_i2] -> Scope3/2
  [pwmSync2] -> Scope3/1, Model2/Trigger
  Model2/2 -> Scope3/4
  [pwmSync3] -> Scope4/1, Model3/Trigger
  Model3/2 -> Scope4/4
  [fb_i3] -> Scope4/2

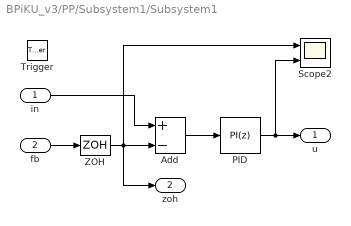
== system BPiKU_v3/PP/Subsystem1/Subsystem1 ==
  in : Inport
  fb : Inport  Port=2
  Trigger : TriggerPort  VariantControl=Variant  PortDimensions=1
  Add : Sum  Inputs=+-
  PID : simulink/Continuous/PID Controller  Controller=PI  Form=Parallel  TimeDomain=Discrete-time  SampleTime=-1  IntegratorMethod=Forward Euler  FilterMethod=Forward Euler  ControllerParametersSource=internal  P=i_kt_p  I=i_kt_int  D=0  UseFilter=on  N=100  TunerSelectOption=Transfer Function Based (PID Tuner App)  InitialConditionSource=internal  InitialConditionForIntegrator=0  InitialConditionForFilter=0  DifferentiatorICPrevScaledInput=0  ExternalReset=none  TrackingMode=off  Kt=1  LimitOutput=on  UpperSaturationLimit=1  LowerSaturationLimit=0  LinearizeAsGain=on  AntiWindupMode=none  Kb=1  POutMin=[]  POutMax=[]  IOutMin=[]  IOutMax=[]  DOutMin=[]  DOutMax=[]  NOutMin=[]  NOutMax=[]  SumOutMin=[]  SumOutMax=[]  SaturationOutMin=[]  SaturationOutMax=[]  PParamMin=[]  PParamMax=[]  IParamMin=[]  IParamMax=[]  DParamMin=[]  DParamMax=[]  NParamMin=[]  NParamMax=[]  KbParamMin=[]  KbParamMax=[]  KtParamMin=[]  KtParamMax=[]  KbOutMin=[]  KbOutMax=[]  KtOutMin=[]  KtOutMax=[]  IntegratorOutMin=[]  IntegratorOutMax=[]  FilterOutMin=[]  FilterOutMax=[]  SumI1OutMin=[]  SumI1OutMax=[]  SumI2OutMin=[]  SumI2OutMax=[]  SumI3OutMin=[]  SumI3OutMax=[]  SumI4OutMin=[]  SumI4OutMax=[]  SumDOutMin=[]  SumDOutMax=[]  DifferentiatorOutMin=[]  DifferentiatorOutMax=[]  FilterDiffOutCoefMin=[]  FilterDiffOutCoefMax=[]  ReciprocalOutMin=[]  ReciprocalOutMax=[]  SumDenOutMin=[]  SumDenOutMax=[]  SumNumOutMin=[]  SumNumOutMax=[]  DivideOutMin=[]  DivideOutMax=[]  IntegratorContinuousStateAttributes=''  IntegratorStateMustResolveToSignalObject=off  IntegratorRTWStateStorageClass=Auto  FilterContinuousStateAttributes=''  FilterStateMustResolveToSignalObject=off  FilterRTWStateStorageClass=Auto  ParallelPVariant=InternalParameters  IdealPVariant=Disabled  IVariant=InternalParameters  DVariant=Disabled  IntegratorVariant=Discrete  SatVariant=Enabled  AWVariant=Passthrough  PCopyVariant=Disabled  TRVariant=Disabled  FdbkBlocksVariant=Forward  IdealPFdbkVariant=Disabled  SatFdbkVariant=Disabled  DerivativeFilterVariant=Disabled  NVariant=Disabled  NCopyVariant=Disabled_SignalSpec  FilterICVariant=Disabled  IntegratorICVariant=InternalICs  ExternalResetVariant=Disabled  TRSumVariant=Passthrough  SumFdbkVariant=Disabled  SumVariant=Sum_PI
  Scope2 : Scope  NumInputPorts=2
  ZOH : ZeroOrderHold  SampleTime=-1
  u : Outport
  zoh : Outport  Port=2
  wires:
  fb/1 -> ZOH/1
  in/1 -> Add/1
  Add/1 -> PID/1
  PID/1 -> Scope2/2, u/1
  ZOH/1 -> Scope2/1, zoh/1, Add/2

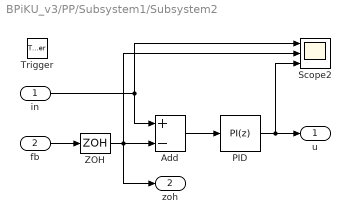
== system BPiKU_v3/PP/Subsystem1/Subsystem2 ==
  in : Inport
  fb : Inport  Port=2
  Trigger : TriggerPort  VariantControl=Variant  PortDimensions=1
  Add : Sum  Inputs=+-
  PID : simulink/Continuous/PID Controller  Controller=PI  Form=Parallel  TimeDomain=Discrete-time  SampleTime=-1  IntegratorMethod=Forward Euler  FilterMethod=Forward Euler  ControllerParametersSource=internal  P=i_kt_p  I=i_kt_int  D=0  UseFilter=on  N=100  TunerSelectOption=Transfer Function Based (PID Tuner App)  InitialConditionSource=internal  InitialConditionForIntegrator=0  InitialConditionForFilter=0  DifferentiatorICPrevScaledInput=0  ExternalReset=none  TrackingMode=off  Kt=1  LimitOutput=on  UpperSaturationLimit=1  LowerSaturationLimit=0  LinearizeAsGain=on  AntiWindupMode=none  Kb=1  POutMin=[]  POutMax=[]  IOutMin=[]  IOutMax=[]  DOutMin=[]  DOutMax=[]  NOutMin=[]  NOutMax=[]  SumOutMin=[]  SumOutMax=[]  SaturationOutMin=[]  SaturationOutMax=[]  PParamMin=[]  PParamMax=[]  IParamMin=[]  IParamMax=[]  DParamMin=[]  DParamMax=[]  NParamMin=[]  NParamMax=[]  KbParamMin=[]  KbParamMax=[]  KtParamMin=[]  KtParamMax=[]  KbOutMin=[]  KbOutMax=[]  KtOutMin=[]  KtOutMax=[]  IntegratorOutMin=[]  IntegratorOutMax=[]  FilterOutMin=[]  FilterOutMax=[]  SumI1OutMin=[]  SumI1OutMax=[]  SumI2OutMin=[]  SumI2OutMax=[]  SumI3OutMin=[]  SumI3OutMax=[]  SumI4OutMin=[]  SumI4OutMax=[]  SumDOutMin=[]  SumDOutMax=[]  DifferentiatorOutMin=[]  DifferentiatorOutMax=[]  FilterDiffOutCoefMin=[]  FilterDiffOutCoefMax=[]  ReciprocalOutMin=[]  ReciprocalOutMax=[]  SumDenOutMin=[]  SumDenOutMax=[]  SumNumOutMin=[]  SumNumOutMax=[]  DivideOutMin=[]  DivideOutMax=[]  IntegratorContinuousStateAttributes=''  IntegratorStateMustResolveToSignalObject=off  IntegratorRTWStateStorageClass=Auto  FilterContinuousStateAttributes=''  FilterStateMustResolveToSignalObject=off  FilterRTWStateStorageClass=Auto  ParallelPVariant=InternalParameters  IdealPVariant=Disabled  IVariant=InternalParameters  DVariant=Disabled  IntegratorVariant=Discrete  SatVariant=Enabled  AWVariant=Passthrough  PCopyVariant=Disabled  TRVariant=Disabled  FdbkBlocksVariant=Forward  IdealPFdbkVariant=Disabled  SatFdbkVariant=Disabled  DerivativeFilterVariant=Disabled  NVariant=Disabled  NCopyVariant=Disabled_SignalSpec  FilterICVariant=Disabled  IntegratorICVariant=InternalICs  ExternalResetVariant=Disabled  TRSumVariant=Passthrough  SumFdbkVariant=Disabled  SumVariant=Sum_PI
  Scope2 : Scope  NumInputPorts=3
  ZOH : ZeroOrderHold  SampleTime=-1
  u : Outport
  zoh : Outport  Port=2
  wires:
  fb/1 -> ZOH/1
  in/1 -> Scope2/1, Add/1
  Add/1 -> PID/1
  PID/1 -> Scope2/3, u/1
  ZOH/1 -> Scope2/2, zoh/1, Add/2

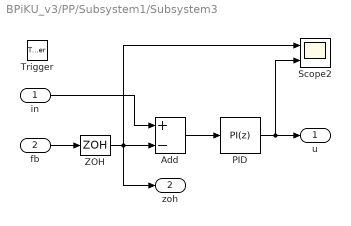
== system BPiKU_v3/PP/Subsystem1/Subsystem3 ==
  in : Inport
  fb : Inport  Port=2
  Trigger : TriggerPort  VariantControl=Variant  PortDimensions=1
  Add : Sum  Inputs=+-
  PID : simulink/Continuous/PID Controller  Controller=PI  Form=Parallel  TimeDomain=Discrete-time  SampleTime=-1  IntegratorMethod=Forward Euler  FilterMethod=Forward Euler  ControllerParametersSource=internal  P=i_kt_p  I=i_kt_int  D=0  UseFilter=on  N=100  TunerSelectOption=Transfer Function Based (PID Tuner App)  InitialConditionSource=internal  InitialConditionForIntegrator=0  InitialConditionForFilter=0  DifferentiatorICPrevScaledInput=0  ExternalReset=none  TrackingMode=off  Kt=1  LimitOutput=on  UpperSaturationLimit=1  LowerSaturationLimit=0  LinearizeAsGain=on  AntiWindupMode=none  Kb=1  POutMin=[]  POutMax=[]  IOutMin=[]  IOutMax=[]  DOutMin=[]  DOutMax=[]  NOutMin=[]  NOutMax=[]  SumOutMin=[]  SumOutMax=[]  SaturationOutMin=[]  SaturationOutMax=[]  PParamMin=[]  PParamMax=[]  IParamMin=[]  IParamMax=[]  DParamMin=[]  DParamMax=[]  NParamMin=[]  NParamMax=[]  KbParamMin=[]  KbParamMax=[]  KtParamMin=[]  KtParamMax=[]  KbOutMin=[]  KbOutMax=[]  KtOutMin=[]  KtOutMax=[]  IntegratorOutMin=[]  IntegratorOutMax=[]  FilterOutMin=[]  FilterOutMax=[]  SumI1OutMin=[]  SumI1OutMax=[]  SumI2OutMin=[]  SumI2OutMax=[]  SumI3OutMin=[]  SumI3OutMax=[]  SumI4OutMin=[]  SumI4OutMax=[]  SumDOutMin=[]  SumDOutMax=[]  DifferentiatorOutMin=[]  DifferentiatorOutMax=[]  FilterDiffOutCoefMin=[]  FilterDiffOutCoefMax=[]  ReciprocalOutMin=[]  ReciprocalOutMax=[]  SumDenOutMin=[]  SumDenOutMax=[]  SumNumOutMin=[]  SumNumOutMax=[]  DivideOutMin=[]  DivideOutMax=[]  IntegratorContinuousStateAttributes=''  IntegratorStateMustResolveToSignalObject=off  IntegratorRTWStateStorageClass=Auto  FilterContinuousStateAttributes=''  FilterStateMustResolveToSignalObject=off  FilterRTWStateStorageClass=Auto  ParallelPVariant=InternalParameters  IdealPVariant=Disabled  IVariant=InternalParameters  DVariant=Disabled  IntegratorVariant=Discrete  SatVariant=Enabled  AWVariant=Passthrough  PCopyVariant=Disabled  TRVariant=Disabled  FdbkBlocksVariant=Forward  IdealPFdbkVariant=Disabled  SatFdbkVariant=Disabled  DerivativeFilterVariant=Disabled  NVariant=Disabled  NCopyVariant=Disabled_SignalSpec  FilterICVariant=Disabled  IntegratorICVariant=InternalICs  ExternalResetVariant=Disabled  TRSumVariant=Passthrough  SumFdbkVariant=Disabled  SumVariant=Sum_PI
  Scope2 : Scope  NumInputPorts=2
  ZOH : ZeroOrderHold  SampleTime=-1
  u : Outport
  zoh : Outport  Port=2
  wires:
  fb/1 -> ZOH/1
  in/1 -> Add/1
  Add/1 -> PID/1
  PID/1 -> Scope2/2, u/1
  ZOH/1 -> Scope2/1, zoh/1, Add/2

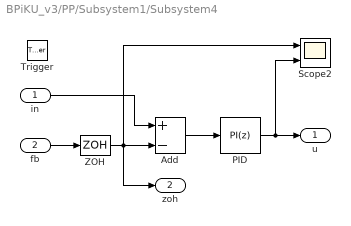
== system BPiKU_v3/PP/Subsystem1/Subsystem4 ==
  in : Inport
  fb : Inport  Port=2
  Trigger : TriggerPort  VariantControl=Variant  PortDimensions=1
  Add : Sum  Inputs=+-
  PID : simulink/Continuous/PID Controller  Controller=PI  Form=Parallel  TimeDomain=Discrete-time  SampleTime=-1  IntegratorMethod=Forward Euler  FilterMethod=Forward Euler  ControllerParametersSource=internal  P=u_k_p  I=u_k_int  D=0  UseFilter=on  N=100  TunerSelectOption=Transfer Function Based (PID Tuner App)  InitialConditionSource=internal  InitialConditionForIntegrator=0  InitialConditionForFilter=0  DifferentiatorICPrevScaledInput=0  ExternalReset=none  TrackingMode=off  Kt=1  LimitOutput=on  UpperSaturationLimit=1  LowerSaturationLimit=0  LinearizeAsGain=on  AntiWindupMode=none  Kb=1  POutMin=[]  POutMax=[]  IOutMin=[]  IOutMax=[]  DOutMin=[]  DOutMax=[]  NOutMin=[]  NOutMax=[]  SumOutMin=[]  SumOutMax=[]  SaturationOutMin=[]  SaturationOutMax=[]  PParamMin=[]  PParamMax=[]  IParamMin=[]  IParamMax=[]  DParamMin=[]  DParamMax=[]  NParamMin=[]  NParamMax=[]  KbParamMin=[]  KbParamMax=[]  KtParamMin=[]  KtParamMax=[]  KbOutMin=[]  KbOutMax=[]  KtOutMin=[]  KtOutMax=[]  IntegratorOutMin=[]  IntegratorOutMax=[]  FilterOutMin=[]  FilterOutMax=[]  SumI1OutMin=[]  SumI1OutMax=[]  SumI2OutMin=[]  SumI2OutMax=[]  SumI3OutMin=[]  SumI3OutMax=[]  SumI4OutMin=[]  SumI4OutMax=[]  SumDOutMin=[]  SumDOutMax=[]  DifferentiatorOutMin=[]  DifferentiatorOutMax=[]  FilterDiffOutCoefMin=[]  FilterDiffOutCoefMax=[]  ReciprocalOutMin=[]  ReciprocalOutMax=[]  SumDenOutMin=[]  SumDenOutMax=[]  SumNumOutMin=[]  SumNumOutMax=[]  DivideOutMin=[]  DivideOutMax=[]  IntegratorContinuousStateAttributes=''  IntegratorStateMustResolveToSignalObject=off  IntegratorRTWStateStorageClass=Auto  FilterContinuousStateAttributes=''  FilterStateMustResolveToSignalObject=off  FilterRTWStateStorageClass=Auto  ParallelPVariant=InternalParameters  IdealPVariant=Disabled  IVariant=InternalParameters  DVariant=Disabled  IntegratorVariant=Discrete  SatVariant=Enabled  AWVariant=Passthrough  PCopyVariant=Disabled  TRVariant=Disabled  FdbkBlocksVariant=Forward  IdealPFdbkVariant=Disabled  SatFdbkVariant=Disabled  DerivativeFilterVariant=Disabled  NVariant=Disabled  NCopyVariant=Disabled_SignalSpec  FilterICVariant=Disabled  IntegratorICVariant=InternalICs  ExternalResetVariant=Disabled  TRSumVariant=Passthrough  SumFdbkVariant=Disabled  SumVariant=Sum_PI
  Scope2 : Scope  NumInputPorts=2
  ZOH : ZeroOrderHold  SampleTime=-1
  u : Outport
  zoh : Outport  Port=2
  wires:
  fb/1 -> ZOH/1
  in/1 -> Add/1
  Add/1 -> PID/1
  PID/1 -> Scope2/2, u/1
  ZOH/1 -> Scope2/1, zoh/1, Add/2
